simulink model "Autopilot_testHarness"  (R2012b)
settings: Solver=ode45  StartTime=0.0  StopTime=10.0  RelTol=1e-3
settings Model: Creator=ssauvage  LastModifiedBy=ssauvage

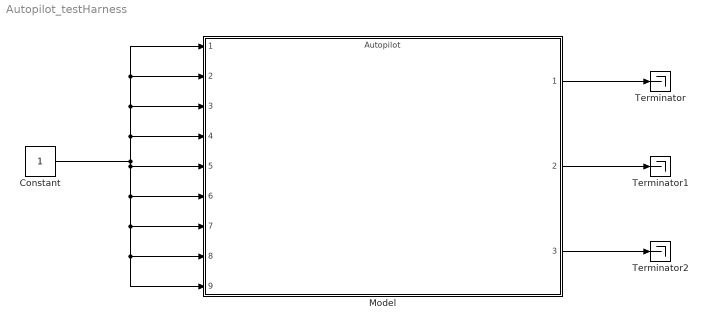
== system Autopilot_testHarness ==
  Constant : Constant
  Model : ModelReference  ModelNameDialog=Autopilot  SimulationMode=Normal  ModelReferenceVersion=1.154  CopyOfModelName=Autopilot  DefaultDataLogging=on
  Terminator : Terminator
  Terminator1 : Terminator
  Terminator2 : Terminator
  wires:
  Constant/1 -> Model/9, Model/8, Model/7, Model/6, Model/5, Model/4, Model/3, Model/2, Model/1
  Model/3 -> Terminator2/1
  Model/2 -> Terminator1/1
  Model/1 -> Terminator/1
